simulink model "P1_Ex2"  (R2018a)
settings: Solver=FixedStepAuto  StartTime=0.0  StopTime=10  RelTol=1e-3  EnableMultiTasking=on
undefined symbols (not defined in the file): Tg, Vmax, Vmin
libraries: arduinolib x2
settings Model: SimulationMode=external  ExtModeTrigDuration=2  Creator=Eneko Lerma  LastModifiedBy=Eneko Lerma
settings OptimizationCC: EnhancedBackFolding=on  PassReuseOutputArgsAs=Individual arguments  MaxStackSize=64  OptimizeBlockOrder=speed  DifferentSizesBufferReuse=on  OptimizationCustomize=off
settings DebuggingCC: ParameterPrecisionLossMsg=none  ParameterTunabilityLossMsg=error
settings HardwareCC: ProdBitPerPointer=32  ProdBitPerSizeT=32  ProdBitPerPtrDiffT=32  ProdLargestAtomicInteger=Long  ProdLargestAtomicFloat=Double  ProdWordSize=32  ProdHWDeviceType=ARM Compatible->ARM Cortex
settings SFSimCC: MATLABDynamicMemAlloc=off
settings RTWCC: SystemTargetFile=ert.tlc  HardwareBoard=Arduino Due  TLCOptions=-aInlineSetEventsForThisBaseRateFcn=TLC_FALSE -aSuppressMultiTaskScheduler=TLC_FALSE -aRateBasedStepFcn=1  TemplateMakefile=ert_default_tmf  GenerateReport=on  Toolchain=Arduino ARM  BuildConfiguration=Faster Runs  IncludeHyperlinkInReport=on  LaunchReport=on  GenerateTraceInfo=on  GenerateTraceReport=on  GenerateTraceReportSl=on  GenerateTraceReportSf=on  GenerateTraceReportEml=on
settings CodeAppCC: ForceParamTrailComments=on  IgnoreCustomStorageClasses=off  OperatorAnnotations=on  SimulinkDataObjDesc=on  SFDataObjDesc=on  InsertBlockDesc=on
settings ERTTargetCC: SupportContinuousTime=on  SupportVariableSizeSignals=on

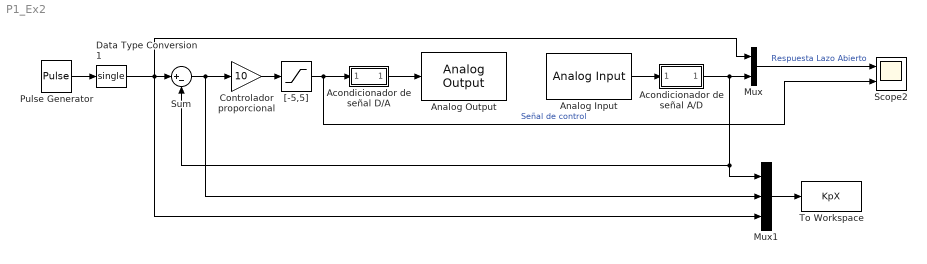
== system P1_Ex2 ==
  Acondicionador de señal A/D : Subsystem
  Acondicionador de señal D/A : Subsystem
  Analog Input : arduinolib/Analog Input  pinNumber=2  ReadResultsOnly=off  ConversionTriggerSource=Software  ExternalTriggerType=uint32(0)  OutputDataType=uint16  EnableConversionCompleteNotify=off  EnableOuputStatus=off  SampleTime=Tg  blockPlatform=arduino
  Analog Output : arduinolib/Analog Output  DACpin=DAC1  blockPlatform=arduino
      settings: SourceProductName=Simulink Support Package for Arduino Hardware  SourceProductBaseCode=ARDUINO
  Controlador proporcional : Gain  Gain=10
  Data Type Conversion1 : DataTypeConversion  OutDataTypeStr=single
  Mux : Mux  Inputs=2
  Mux1 : Mux  Inputs=3
  Pulse Generator : DiscretePulseGenerator  PulseType=Time based  Amplitude=2  Period=5  PulseWidth=50  SampleTime=0.005
  Scope2 : Scope  NumInputPorts=2
  Sum : Sum  Inputs=|+-
  To Workspace : ToWorkspace  VariableName=KpX  SaveFormat=Structure With Time  SampleTime=-1
  "[-5,5]" : Saturate  UpperLimit=Vmax  LowerLimit=Vmin  OutDataTypeStr=single
  wires:
  Mux/1 -> Scope2/1  "Respuesta Lazo Abierto"
  "[-5,5]"/1 -> Scope2/2, Acondicionador de señal D/A/1("  ")  "Señal de control"
  Acondicionador de señal D/A/1(" ") -> Analog Output/1
  Pulse Generator/1 -> Data Type Conversion1/1
  Analog Input/1 -> Acondicionador de señal A/D/1(" ")
  Acondicionador de señal A/D/1(" ") -> Sum/2, Mux1/1, Mux/2
  Data Type Conversion1/1 -> Mux1/3, Sum/1, Mux/1
  Sum/1 -> Controlador proporcional/1, Mux1/2
  Controlador proporcional/1 -> "[-5,5]"/1
  Mux1/1 -> To Workspace/1

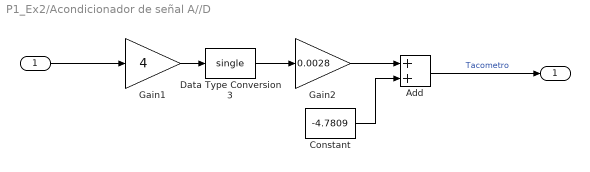
== system P1_Ex2/Acondicionador de señal A//D ==
  " " : Inport
  Add : Sum  AccumDataTypeStr=single
  Constant : Constant  Value=-4.7809  OutDataTypeStr=single
  Data Type Conversion3 : DataTypeConversion  OutDataTypeStr=single
  Gain1 : Gain  Gain=4  OutDataTypeStr=uint16
  Gain2 : Gain  Gain=0.0028  OutDataTypeStr=single
  " " : Outport
  wires:
  Gain1/1 -> Data Type Conversion3/1
  " "/1 -> Gain1/1
  Add/1 -> " "/1  "Tacometro"
  Gain2/1 -> Add/1
  Constant/1 -> Add/2
  Data Type Conversion3/1 -> Gain2/1

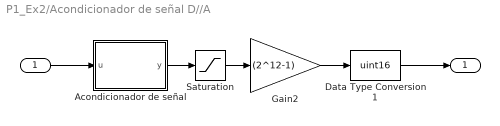
== system P1_Ex2/Acondicionador de señal D//A ==
  "  " : Inport  OutDataTypeStr=single
  Acondicionador de señal : MATLAB Function  TreatAsAtomicUnit=on
  Data Type Conversion1 : DataTypeConversion  OutDataTypeStr=uint16
  Gain2 : Gain  Gain=(2^12-1)  OutDataTypeStr=single
  Saturation : Saturate  UpperLimit=1  LowerLimit=0  OutDataTypeStr=single
  " " : Outport  OutDataTypeStr=uint16
  wires:
  Saturation/1 -> Gain2/1
  Data Type Conversion1/1 -> " "/1
  Acondicionador de señal/1(y) -> Saturation/1
  "  "/1 -> Acondicionador de señal/1(u)
  Gain2/1 -> Data Type Conversion1/1

== matlab function P1_Ex2/Acondicionador de señal D//A/Acondicionador de señal ==
  data: u input; y output
function y = fcn(u)
y =0.1342*u+0.3926;
